simulink model "DWT(ALIAS)"  (R2016a)
settings: Solver=VariableStepAuto  StartTime=0.0  StopTime=4000  RelTol=1e-3
libraries: dspsrcs4 x1
settings Model: Creator=HP  LastModifiedBy=HP

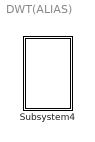
== system DWT(ALIAS) ==
  Subsystem4 : Subsystem

== system DWT(ALIAS)/Subsystem4 ==
  Subsystem4 : Subsystem

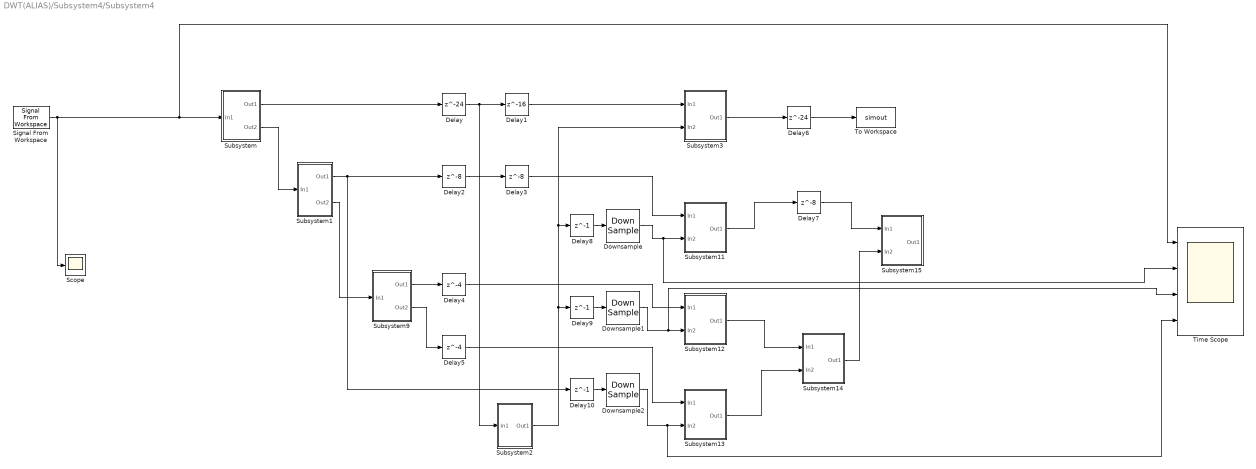
== system DWT(ALIAS)/Subsystem4/Subsystem4 ==
  Delay : Delay  DelayLength=24  InitialCondition=0  InputProcessing=Columns as channels (frame based)
  Delay1 : Delay  DelayLength=16  InitialCondition=0  InputProcessing=Columns as channels (frame based)
  Delay10 : Delay  DelayLength=1  InitialCondition=0
  Delay2 : Delay  DelayLength=8  InitialCondition=0  InputProcessing=Columns as channels (frame based)
  Delay3 : Delay  DelayLength=8  InitialCondition=0
  Delay4 : Delay  DelayLength=4  InitialCondition=0
  Delay5 : Delay  DelayLength=4  InitialCondition=0
  Delay6 : Delay  DelayLength=24  InitialCondition=0  InputProcessing=Columns as channels (frame based)
  Delay7 : Delay  DelayLength=8  InitialCondition=0  InputProcessing=Columns as channels (frame based)
  Delay8 : Delay  DelayLength=1  InitialCondition=0
  Delay9 : Delay  DelayLength=1  InitialCondition=0
  Downsample : DownSample  RateOptions=Allow multirate processing  ic=-1
  Downsample1 : DownSample  N=4  RateOptions=Allow multirate processing  ic=-1
  Downsample2 : DownSample  N=8  phase=1  RateOptions=Allow multirate processing  ic=-1
  Scope : Scope
  Signal From Workspace : dspsrcs4/Signal From Workspace  X=y  Ts=1  nsamps=1  OutputAfterFinalValue=Setting to zero  ignoreOrWarnInputAndFrameLengths=off  OutputFrames=off
  Subsystem : Subsystem
  Subsystem1 : Subsystem
  Subsystem11 : Subsystem
  Subsystem12 : Subsystem
  Subsystem13 : Subsystem
  Subsystem14 : Subsystem
  Subsystem15 : Subsystem
  Subsystem2 : Subsystem
  Subsystem3 : Subsystem
  Subsystem9 : Subsystem
  Time Scope : Scope  NumInputPorts=4
  To Workspace : ToWorkspace  VariableName=simout  SaveFormat=Timeseries  SampleTime=-1
  wires:
  Subsystem1/2(Out2) -> Subsystem9/1(In1)
  Delay3/1 -> Subsystem11/1(In1)
  Downsample/1 -> Time Scope/2, Subsystem11/2(In2)
  Subsystem9/1(Out1) -> Delay4/1
  Subsystem/1(Out1) -> Delay/1
  Signal From Workspace/1 -> Scope/1, Time Scope/1, Subsystem/1(In1)
  Subsystem/2(Out2) -> Subsystem1/1(In1)
  Delay2/1 -> Delay3/1
  Subsystem11/1(Out1) -> Delay7/1
  Delay1/1 -> Subsystem3/1(In1)
  Delay/1 -> Subsystem2/1(In1), Delay1/1
  Delay4/1 -> Subsystem12/1(In1)
  Downsample2/1 -> Time Scope/4, Subsystem13/2(In2)
  Subsystem13/1(Out1) -> Subsystem14/2(In2)
  Subsystem3/1(Out1) -> Delay6/1
  Subsystem1/1(Out1) -> Delay2/1, Delay10/1
  Subsystem14/1(Out1) -> Subsystem15/2(In2)
  Subsystem9/2(Out2) -> Delay5/1
  Downsample1/1 -> Time Scope/3, Subsystem12/2(In2)
  Delay5/1 -> Subsystem13/1(In1)
  Subsystem12/1(Out1) -> Subsystem14/1(In1)
  Delay7/1 -> Subsystem15/1(In1)
  Subsystem2/1(Out1) -> Delay9/1, Subsystem3/2(In2), Delay8/1
  Delay8/1 -> Downsample/1
  Delay9/1 -> Downsample1/1
  Delay10/1 -> Downsample2/1
  Delay6/1 -> To Workspace/1

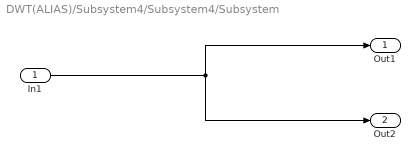
== system DWT(ALIAS)/Subsystem4/Subsystem4/Subsystem ==
  In1 : Inport
  Out1 : Outport
  Out2 : Outport  Port=2
  wires:
  In1/1 -> Out1/1, Out2/1

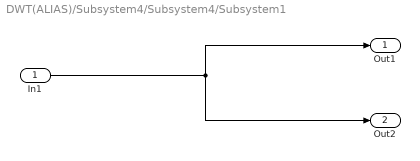
== system DWT(ALIAS)/Subsystem4/Subsystem4/Subsystem1 ==
  In1 : Inport
  Out1 : Outport
  Out2 : Outport  Port=2
  wires:
  In1/1 -> Out1/1, Out2/1

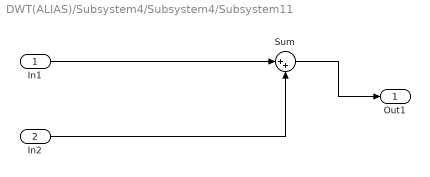
== system DWT(ALIAS)/Subsystem4/Subsystem4/Subsystem11 ==
  In1 : Inport
  In2 : Inport  Port=2
  Sum : Sum  Inputs=|++
  Out1 : Outport
  wires:
  In1/1 -> Sum/1
  In2/1 -> Sum/2
  Sum/1 -> Out1/1

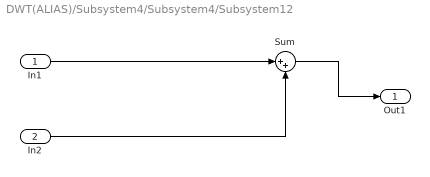
== system DWT(ALIAS)/Subsystem4/Subsystem4/Subsystem12 ==
  In1 : Inport
  In2 : Inport  Port=2
  Sum : Sum  Inputs=|++
  Out1 : Outport
  wires:
  In1/1 -> Sum/1
  In2/1 -> Sum/2
  Sum/1 -> Out1/1

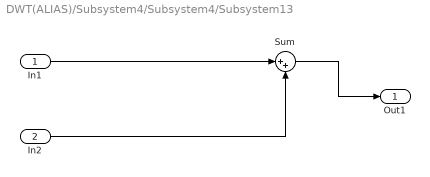
== system DWT(ALIAS)/Subsystem4/Subsystem4/Subsystem13 ==
  In1 : Inport
  In2 : Inport  Port=2
  Sum : Sum  Inputs=|++
  Out1 : Outport
  wires:
  In1/1 -> Sum/1
  In2/1 -> Sum/2
  Sum/1 -> Out1/1

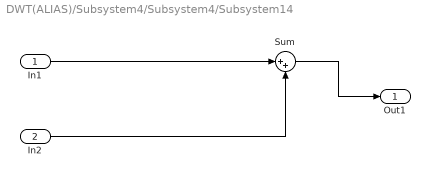
== system DWT(ALIAS)/Subsystem4/Subsystem4/Subsystem14 ==
  In1 : Inport
  In2 : Inport  Port=2
  Sum : Sum  Inputs=|++
  Out1 : Outport
  wires:
  In1/1 -> Sum/1
  In2/1 -> Sum/2
  Sum/1 -> Out1/1

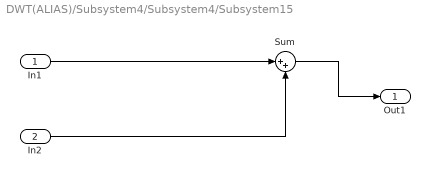
== system DWT(ALIAS)/Subsystem4/Subsystem4/Subsystem15 ==
  In1 : Inport
  In2 : Inport  Port=2
  Sum : Sum  Inputs=|++
  Out1 : Outport
  wires:
  In1/1 -> Sum/1
  In2/1 -> Sum/2
  Sum/1 -> Out1/1

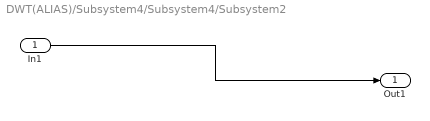
== system DWT(ALIAS)/Subsystem4/Subsystem4/Subsystem2 ==
  In1 : Inport
  Out1 : Outport
  wires:
  In1/1 -> Out1/1

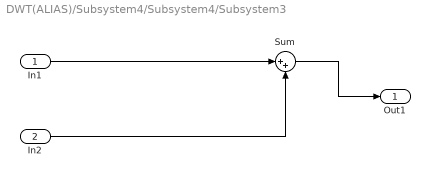
== system DWT(ALIAS)/Subsystem4/Subsystem4/Subsystem3 ==
  In1 : Inport
  In2 : Inport  Port=2
  Sum : Sum  Inputs=|++
  Out1 : Outport
  wires:
  In1/1 -> Sum/1
  In2/1 -> Sum/2
  Sum/1 -> Out1/1

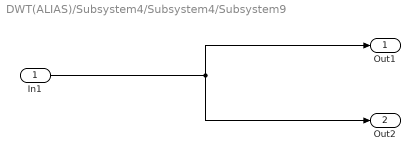
== system DWT(ALIAS)/Subsystem4/Subsystem4/Subsystem9 ==
  In1 : Inport
  Out1 : Outport
  Out2 : Outport  Port=2
  wires:
  In1/1 -> Out1/1, Out2/1
